simulink model "soc_dvbs2_fpga"  (R2025b)
settings: Solver=FixedStepDiscrete  StartTime=0.0  StopTime=0  RelTol=1e-3
InitFcn:
  | soc_dvbs2_init;
values from neighbouring files (symbols this model uses):
  Rsym = 4e6    (= 4000000)    [soc_dvbs2_init.m]
  soc_dvbs2_txPacketBits = [1 1 0 1 0 1 1 1 0 1 1 1 ... (2972 elements, 2972x1)]    [soc_dvbs2_txPacketBits.mat]
  syncWord = (dec2bin(hex2dec('AC')) - '0').'    [soc_dvbs2_init.m]
  txDataOut = txobj(frameBits(:))    [soc_dvbs2_init.m]
  txFiltCoeff = txobj.pTxFilterCoeff    [soc_dvbs2_init.m]
undefined symbols (not defined in the file or in its folder): Add, coefficientsLog, coefficientsSqrt1, coefficientsSqrt2, dataBits, designMultirateFIR, noisePow, NumBits1, NumBits2, seedsURNG1, seedsURNG2, Shift, Slope1, Slope2, soc_dvbs2_designFIRFilter, txDataOutS1, txDataOutS10, txDataOutS12, txDataOutS13, txDataOutS14, txDataOutS15, txDataOutS16, txDataOutS18, txDataOutS19, txDataOutS2, txDataOutS20, txDataOutS21, txDataOutS22, txDataOutS24, txDataOutS25, txDataOutS26, txDataOutS27, txDataOutS3, txDataOutS4, txDataOutS5, txDataOutS6, txDataOutS7, txDataOutS8, txDataOutS9
libraries: simulink x214, hdlsllib x211, dspsigops x22, dsphdlfiltering2 x8, dsphdlsigops2 x5, commseqgen3 x5, dsphdlmathfun2 x3, hwlogicconnlib x2, whdledac x2, commhdlcrc x2, whdlutilities x1, whdlmod x1
(part 4 of 12)

== system soc_dvbs2_fpga/DVBS2/DVBS2 TxRx/DVB-S2 HDL Receiver/Synchronizer and PL Header Decoder/Fine Phase Synchronizer/Direct Digital Synthesis ==
  v : Inport
  rst : Inport  Port=2
  Constant : Constant  Value=true  SampleTime=-1
  Constant1 : Constant  Value=FPCV  OutDataTypeStr=boolean  SampleTime=-1
  Constant2 : Constant  Value=complex(1)  OutDataTypeStr=Inherit: Inherit via back propagation  SampleTime=-1
  Data Type Conversion : DataTypeConversion  OutDataTypeStr=fixdt(1,21,21)  SaturateOnIntegerOverflow=off  RndMeth=Floor
  Data Type Conversion1 : DataTypeConversion  OutDataTypeStr=fixdt(1,21,0)  ConvertRealWorld=Stored Integer (SI)  SaturateOnIntegerOverflow=off  RndMeth=Floor
  Delay1 : Delay  DelayLength=1
  Delay12 : Delay  DelayLength=1
  Multiport Switch : MultiPortSwitch  DataPortOrder=Zero-based contiguous  Inputs=2  zeroidx=on  SaturateOnIntegerOverflow=off  InputSameDT=off
  NCO HDL Optimized : dsphdlsigops2/NCO  PhaseIncrementSource=Property  PhaseIncrement=0  PhaseOffsetSource=Input port  PhaseOffset=0  DitherSource=None  NumDitherBits=4  SamplesPerFrame=1  LUTCompress=off  ResetAction=on  Waveform=Complex exponential  PhasePort=off  SimulateUsing=Code generation  AccumulatorWL=21  PhaseQuantization=on  NumQuantizerAccumulatorBits=14  OutputDataType=Binary point scaling  OutputWL=16  OutputFL=14
  Terminator : Terminator
  xph : Outport
  wires:
  rst/1 -> NCO HDL Optimized/2
  Multiport Switch/1 -> Delay1/1
  Constant2/1 -> Multiport Switch/2
  Constant1/1 -> Multiport Switch/1
  Delay1/1 -> xph/1
  Delay12/1 -> Data Type Conversion/1
  NCO HDL Optimized/2 -> Terminator/1
  Constant/1 -> NCO HDL Optimized/3
  NCO HDL Optimized/1 -> Multiport Switch/3
  Data Type Conversion1/1 -> NCO HDL Optimized/1
  Data Type Conversion/1 -> Data Type Conversion1/1
  v/1 -> Delay12/1

== system soc_dvbs2_fpga/DVBS2/DVBS2 TxRx/DVB-S2 HDL Receiver/Synchronizer and PL Header Decoder/Fine Phase Synchronizer/Loop Filter ==
  e : Inport
  En : Inport  Port=2
  rst : Inport  Port=3
  Add : Sum  Inputs=|++  OutDataTypeStr=Inherit: Same as first input
  Delay1 : Delay
  Delay12 : Delay
  Gain : Gain  Gain=fi(config.FPCLoopFilterIntegGain/(2*pi),0,16)  ParamDataTypeStr=Inherit: Inherit from 'Gain'  OutDataTypeStr=fixdt(1,21,21)
  Unit Delay Enabled Resettable Synchronous : hdlsllib/Discrete/Unit Delay Enabled Resettable Synchronous  InitialCondition=0.0  SampleTime=-1
  v : Outport
  rstOut : Outport  Port=2
  wires:
  rst/1 -> Unit Delay Enabled Resettable Synchronous/3, rstOut/1
  En/1 -> Unit Delay Enabled Resettable Synchronous/2
  Delay1/1 -> Gain/1
  Delay12/1 -> Add/1
  Unit Delay Enabled Resettable Synchronous/1 -> v/1, Add/2
  Add/1 -> Unit Delay Enabled Resettable Synchronous/1
  Gain/1 -> Delay12/1
  e/1 -> Delay1/1

== system soc_dvbs2_fpga/DVBS2/DVBS2 TxRx/DVB-S2 HDL Receiver/Synchronizer and PL Header Decoder/Fine Phase Synchronizer/Phase Error Detector ==
  dataIn : Inport
  Compare To Constant : simulink/Logic and Bit Operations/Compare To Constant  relop=>=  const=0  OutDataTypeStr=boolean
  Compare To Constant1 : simulink/Logic and Bit Operations/Compare To Constant  relop=>=  const=0  OutDataTypeStr=boolean
  Complex to Real-Imag : ComplexToRealImag
  Complex to Real-Imag1 : ComplexToRealImag  Output=Imag
  Constant : Constant  OutDataTypeStr=fixdt(1,2,0)  SampleTime=-1
  Constant1 : Constant  Value=-1  OutDataTypeStr=fixdt(1,2,0)  SampleTime=-1
  Constant2 : Constant  OutDataTypeStr=fixdt(1,2,0)  SampleTime=-1
  Delay{1..5,12} (6 alike) : Delay  DelayLength=1
  Delay6 : Delay
  Delay7 : Delay
  Delay8 : Delay
  Product : Product  OutDataTypeStr=Inherit: Same as first input
  Real-Imag to Complex : RealImagToComplex
  Switch : Switch  Criteria=u2 ~= 0  SaturateOnIntegerOverflow=off  InputSameDT=off
  Switch1 : Switch  Criteria=u2 ~= 0  SaturateOnIntegerOverflow=off  InputSameDT=off
  e : Outport
  wires:
  Delay8/1 -> Complex to Real-Imag1/1
  Delay7/1 -> Product/2
  Delay6/1 -> Product/1
  Delay5/1 -> Delay6/1
  Delay4/1 -> Real-Imag to Complex/2
  Delay3/1 -> Real-Imag to Complex/1
  Delay2/1 -> Compare To Constant1/1
  Delay1/1 -> Delay5/1
  Delay12/1 -> Compare To Constant/1
  Complex to Real-Imag1/1 -> e/1
  Product/1 -> Delay8/1
  dataIn/1 -> Complex to Real-Imag/1, Delay1/1
  Real-Imag to Complex/1 -> Delay7/1
  Switch1/1 -> Delay4/1
  Switch/1 -> Delay3/1
  Constant2/1 -> Switch1/3
  Constant1/1 -> Switch/3, Switch1/1
  Constant/1 -> Switch/1
  Compare To Constant1/1 -> Switch1/2
  Compare To Constant/1 -> Switch/2
  Complex to Real-Imag/2 -> Delay2/1
  Complex to Real-Imag/1 -> Delay12/1

== system soc_dvbs2_fpga/DVBS2/DVBS2 TxRx/DVB-S2 HDL Receiver/Synchronizer and PL Header Decoder/Fine Phase Synchronizer/Power Q and Beta Offset Rotation ==
  dataIn : Inport
  mod : Inport  Port=2
  Complex Multiplier : Subsystem  VariantControl=Use 3 multipliers and 5 adders
      mask Display: disp(['Complex Multiplier' newline 'Latency = 7']);
  Complex Multiplier1 : Subsystem  VariantControl=Use 3 multipliers and 5 adders
      mask Display: disp(['Complex Multiplier' newline 'Latency = 7']);
  Complex Multiplier2 : Subsystem  VariantControl=Use 3 multipliers and 5 adders
      mask Display: disp(['Complex Multiplier' newline 'Latency = 7']);
  Delay{1..3,5,7,9..12,24..27,36} (14 alike) : Delay  DelayLength=1
  Delay{4,6,8,13..20} (11 alike) : Delay  DelayLength=7
  Delay{28..35} (8 alike) : Delay
  Gain : Subsystem  VariantControl=Use 3 multipliers and 5 adders
      mask Display: disp(['Rotate by pi/4' newline 'Latency = 7']);
  Gain1 : Subsystem  VariantControl=Use 3 multipliers and 5 adders
      mask Display: disp(['Rotate by pi/4' newline 'Latency = 7']);
  Multiport Switch : MultiPortSwitch  DataPortOrder=Zero-based contiguous  Inputs=4  zeroidx=on  SaturateOnIntegerOverflow=off  InputSameDT=off
  dataOut : Outport
  wires:
  Delay20/1 -> Delay30/1
  Delay19/1 -> Delay28/1
  Delay36/1 -> dataOut/1
  Delay15/1 -> Delay26/1
  Delay14/1 -> Delay25/1
  Delay13/1 -> Delay24/1
  Delay12/1 -> Complex Multiplier2/2(In2)
  Delay2/1 -> Complex Multiplier1/1(In1)
  Complex Multiplier1/1(Out1) -> Delay10/1
  Delay5/1 -> Complex Multiplier1/2(In2)
  Complex Multiplier/1(Out1) -> Delay2/1, Delay1/1
  mod/1 -> Multiport Switch/1
  Delay35/1 -> Gain1/1(In1)
  Delay34/1 -> Delay20/1
  Delay33/1 -> Gain/1(In1)
  Delay32/1 -> Delay19/1
  Delay31/1 -> Multiport Switch/5
  Delay30/1 -> Multiport Switch/4
  Delay29/1 -> Multiport Switch/3
  Delay28/1 -> Multiport Switch/2
  Delay27/1 -> Delay35/1
  Delay26/1 -> Delay34/1
  Delay25/1 -> Delay33/1
  Delay24/1 -> Delay32/1
  Delay11/1 -> Delay13/1
  Delay9/1 -> Delay14/1
  Delay10/1 -> Delay15/1, Complex Multiplier2/1(In1)
  Delay18/1 -> Delay12/1
  Delay17/1 -> Delay11/1
  Delay16/1 -> Delay9/1
  Delay8/1 -> Delay7/1
  Delay6/1 -> Delay5/1
  Delay4/1 -> Delay3/1
  Delay7/1 -> Delay18/1
  Delay3/1 -> Delay17/1
  Delay1/1 -> Delay16/1
  dataIn/1 -> Delay8/1, Delay6/1, Complex Multiplier/2(In2), Complex Multiplier/1(In1), Delay4/1
  Multiport Switch/1 -> Delay36/1
  Gain/1(Out1) -> Delay29/1
  Gain1/1(Out1) -> Delay31/1
  Complex Multiplier2/1(Out1) -> Delay27/1

== system soc_dvbs2_fpga/DVBS2/DVBS2 TxRx/DVB-S2 HDL Receiver/Synchronizer and PL Header Decoder/PL Header Recovery/No HDL ==
  has Pilots : Inport
  Enable : EnablePort
  To Workspace : ToWorkspace  VariableName=simHasPilots  SaveFormat=Timeseries  SampleTime=-1
      settings: Save2DSignal=2-D array (concatenate along first dimension)
  wires:
  has Pilots/1 -> To Workspace/1

== system soc_dvbs2_fpga/DVBS2/DVBS2 TxRx/DVB-S2 HDL Receiver/Synchronizer and PL Header Decoder/PL Header Recovery/No HDL1 ==
  valid : Inport
  endOfPLSc : Inport  Port=2
  Bias : Bias  Bias=1  SaturateOnIntegerOverflow=off
  Data Type Conversion : DataTypeConversion  OutDataTypeStr=double  SaturateOnIntegerOverflow=off  RndMeth=Floor
  HDL Counter : hdlsllib/Sources/HDL Counter  CountType=Free running  CountInit=0  CountStep=1  CountMax=25  CountFromType=Initial value  CountFrom=0  CountResetPort=off  CountLoadPort=off  CountEnbPort=on  CountDirPort=off  CountHitOutputPort=off  CountDataType=Unsigned  CountWordLen=32  CountFracLen=0  CountSampTime=1
  Subsystem : Subsystem
  wires:
  endOfPLSc/1 -> Subsystem/Enable
  Bias/1 -> Subsystem/1(In1)
  valid/1 -> HDL Counter/1
  Data Type Conversion/1 -> Bias/1
  HDL Counter/1 -> Data Type Conversion/1

== system soc_dvbs2_fpga/DVBS2/DVBS2 TxRx/DVB-S2 HDL Receiver/Synchronizer and PL Header Decoder/PL Header Recovery/PL Frame Demultiplexer ==
  endOfSOFIn : Inport
  validIn : Inport  Port=2
  Compare To Constant : simulink/Logic and Bit Operations/Compare To Constant  relop=<=  const=config.PLSCLength - 1  OutDataTypeStr=boolean
  Delay : Delay  DelayLength=64
  Delay{1..3,5..8,10..13} (11 alike) : Delay  DelayLength=1
  HDL Counter : hdlsllib/Sources/HDL Counter  CountType=Free running  CountInit=0  CountStep=1  CountMax=25  CountFromType=Initial value  CountFrom=0  CountResetPort=on  CountLoadPort=off  CountEnbPort=on  CountDirPort=off  CountHitOutputPort=off  CountDataType=Unsigned  CountWordLen=32  CountFracLen=0  CountSampTime=1
  Logical Operator : Logic  Inputs=3  AllPortsSameDT=off  OutDataTypeStr=boolean
  Logical Operator1 : Logic  AllPortsSameDT=off  OutDataTypeStr=boolean
  Logical Operator2 : Logic  Operator=NOT  AllPortsSameDT=off  OutDataTypeStr=boolean
  Unit Delay Enabled Synchronous : hdlsllib/Discrete/Unit Delay Enabled Synchronous  InitialCondition=0.0  SampleTime=-1
  hValid : Outport
  dValid : Outport  Port=2
  endOfPLSC : Outport  Port=3
  wires:
  Delay/1 -> Delay5/1
  Delay13/1 -> endOfPLSC/1
  Delay12/1 -> dValid/1
  Delay11/1 -> hValid/1
  Delay8/1 -> Logical Operator1/2
  Delay7/1 -> Delay11/1
  Delay6/1 -> Logical Operator2/1
  Delay5/1 -> Delay10/1
  Delay2/1 -> Logical Operator/3, Delay8/1
  Delay1/1 -> Logical Operator/2
  Delay3/1 -> Logical Operator/1
  Delay10/1 -> Delay13/1
  HDL Counter/1 -> Compare To Constant/1
  Logical Operator1/1 -> Delay12/1
  Logical Operator2/1 -> Logical Operator1/1
  Unit Delay Enabled Synchronous/1 -> Delay3/1
  Compare To Constant/1 -> Delay1/1
  Logical Operator/1 -> Delay7/1, Delay6/1
  validIn/1 -> HDL Counter/2, Delay2/1
  endOfSOFIn/1 -> Unit Delay Enabled Synchronous/1, Delay/1, Unit Delay Enabled Synchronous/2, HDL Counter/1

== system soc_dvbs2_fpga/DVBS2/DVBS2 TxRx/DVB-S2 HDL Receiver/Synchronizer and PL Header Decoder/PL Header Recovery/PL Header Decoder ==
  dataIn : Inport
  hasPilots : Inport  Port=2
  endOfSOF : Inport  Port=3
  validIn : Inport  Port=4
  Bit Flipping and Averaging : Subsystem
  Constant : Constant  Value=complex(0)  OutDataTypeStr=Inherit: Inherit via back propagation  SampleTime=-1
  Delay{1..4} (4 alike) : Delay  DelayLength=1
  Delay5 : Delay  DelayLength=10
  Delay6 : Delay  DelayLength=4
  Extract Bits2 : simulink/Logic and Bit Operations/Extract Bits  bitsToExtract=Range of bits  numBits=8  bitIdxRange=[1 5]  outScalingMode=Treat bit field as an integer
  Extract Bits3 : simulink/Logic and Bit Operations/Extract Bits  bitsToExtract=Range of bits  numBits=8  bitIdxRange=0  outScalingMode=Treat bit field as an integer
  ML Decoder : Subsystem
  PLSC Descrambler : Subsystem
  Switch : Switch  Criteria=u2 ~= 0  SaturateOnIntegerOverflow=off  InputSameDT=off
  pi/2 BPSK Soft Bit Generator : Subsystem
  modcod : Outport
  FECFrame : Outport  Port=2
  wires:
  Delay6/1 -> Bit Flipping and Averaging/5(hasPilots)
  Delay5/1 -> Delay6/1
  Delay4/1 -> Delay5/1
  Delay2/1 -> PLSC Descrambler/3(validIn), Switch/2
  Delay1/1 -> PLSC Descrambler/2(resetIn)
  Delay3/1 -> Switch/1
  Bit Flipping and Averaging/3(resetOut) -> ML Decoder/3(reset)
  pi/2 BPSK Soft Bit Generator/4(resetOut) -> Bit Flipping and Averaging/4(resetIn)
  PLSC Descrambler/4(resetOut) -> pi/2 BPSK Soft Bit Generator/4(resetIn)
  Extract Bits2/1 -> modcod/1
  Extract Bits3/1 -> FECFrame/1
  ML Decoder/1(bits6Out) -> Extract Bits2/1, Extract Bits3/1
  Bit Flipping and Averaging/2(validOut) -> ML Decoder/2(PLSCValid32)
  PLSC Descrambler/3(validOut) -> pi/2 BPSK Soft Bit Generator/3(validIn)
  pi/2 BPSK Soft Bit Generator/3(validOut) -> Bit Flipping and Averaging/3(validIn)
  hasPilots/1 -> Delay4/1
  pi/2 BPSK Soft Bit Generator/2(indexIndicatorOut) -> Bit Flipping and Averaging/2(indexIndicater)
  Bit Flipping and Averaging/1(dataOut) -> ML Decoder/1(dataIn)
  Switch/1 -> PLSC Descrambler/1(dataIn)
  Constant/1 -> Switch/3
  PLSC Descrambler/2(indexIndicator) -> pi/2 BPSK Soft Bit Generator/2(indexIndicatorIn)
  PLSC Descrambler/1(dataOut) -> pi/2 BPSK Soft Bit Generator/1(dataIn)
  pi/2 BPSK Soft Bit Generator/1(dataOut) -> Bit Flipping and Averaging/1(dataIn)
  endOfSOF/1 -> Delay1/1
  dataIn/1 -> Delay3/1
  validIn/1 -> Delay2/1

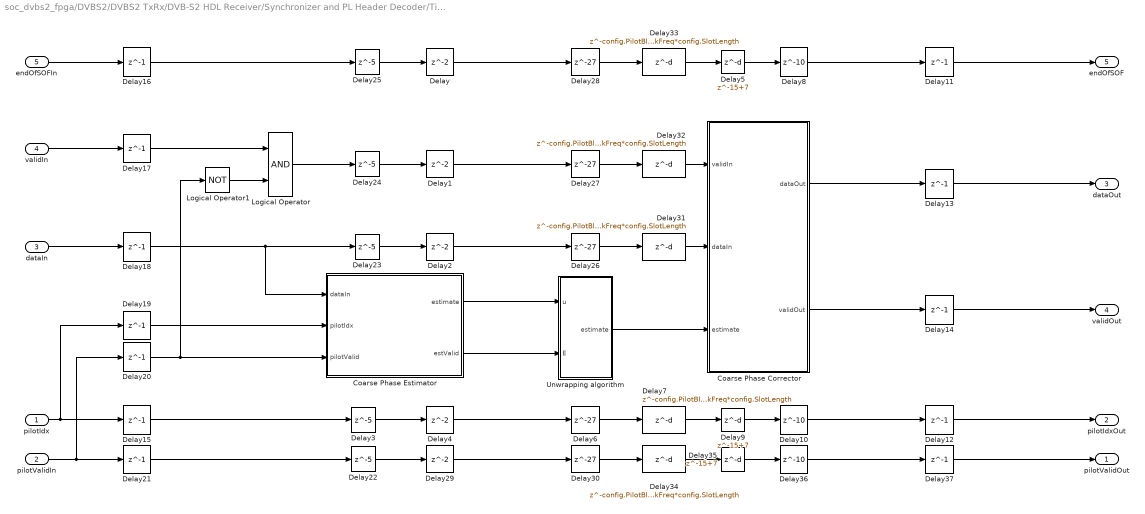
== system soc_dvbs2_fpga/DVBS2/DVBS2 TxRx/DVB-S2 HDL Receiver/Synchronizer and PL Header Decoder/Time Frequency and Coarse Phase Synchronizer/Coarse Phase Synchronizer ==
  pilotIdx : Inport
  pilotValidIn : Inport  Port=2
  dataIn : Inport  Port=3
  validIn : Inport  Port=4
  endOfSOFIn : Inport  Port=5
  Coarse Phase Corrector : Subsystem
  Coarse Phase Estimator : Subsystem
  Delay{,1..2,4,29} (5 alike) : Delay
  Delay10 : Delay  DelayLength=10  InitialCondition=0
  Delay{11..21,37} (12 alike) : Delay  DelayLength=1  InitialCondition=0
  Delay{3,22..25} (5 alike) : Delay  DelayLength=5  InitialCondition=0
  Delay{6,26..28,30} (5 alike) : Delay  DelayLength=27
  Delay{7,31..34} (5 alike) : Delay  DelayLength=config.PilotBlkFreq*config.SlotLength
  Delay35 : Delay  DelayLength=15+7
  Delay36 : Delay  DelayLength=10  InitialCondition=0
  Delay5 : Delay  DelayLength=15+7
  Delay8 : Delay  DelayLength=10  InitialCondition=0
  Delay9 : Delay  DelayLength=15+7
  Logical Operator : Logic  AllPortsSameDT=off  OutDataTypeStr=boolean
  Logical Operator1 : Logic  Operator=NOT  AllPortsSameDT=off  OutDataTypeStr=boolean
  Unwrapping algorithm : Subsystem
      mask init:
      | Simulink.suppressDiagnostic(gcb, 'SimulinkFixedPoint:util:Overflowoccurred');
  pilotValidOut : Outport
  pilotIdxOut : Outport  Port=2
  dataOut : Outport  Port=3
  validOut : Outport  Port=4
  endOfSOF : Outport  Port=5
  wires:
  Delay37/1 -> pilotValidOut/1
  Delay36/1 -> Delay37/1
  Delay35/1 -> Delay36/1
  Delay34/1 -> Delay35/1
  Delay30/1 -> Delay34/1
  Delay29/1 -> Delay30/1
  Delay22/1 -> Delay29/1
  Delay21/1 -> Delay22/1
  Delay15/1 -> Delay3/1
  Delay12/1 -> pilotIdxOut/1
  Delay10/1 -> Delay12/1
  Delay9/1 -> Delay10/1
  Delay7/1 -> Delay9/1
  Delay6/1 -> Delay7/1
  Delay4/1 -> Delay6/1
  Delay3/1 -> Delay4/1
  Logical Operator1/1 -> Logical Operator/2
  Delay17/1 -> Logical Operator/1
  Delay18/1 -> Delay23/1, Coarse Phase Estimator/1(dataIn)
  Coarse Phase Estimator/1(estimate) -> Unwrapping algorithm/1(u)
  Delay33/1 -> Delay5/1
  Delay32/1 -> Coarse Phase Corrector/1(validIn)
  Delay31/1 -> Coarse Phase Corrector/2(dataIn)
  Delay27/1 -> Delay32/1
  Unwrapping algorithm/1(estimate) -> Coarse Phase Corrector/3(estimate)
  Delay28/1 -> Delay33/1
  Delay26/1 -> Delay31/1
  Coarse Phase Estimator/2(estValid) -> Unwrapping algorithm/2(E)
  Coarse Phase Corrector/2(validOut) -> Delay14/1
  Coarse Phase Corrector/1(dataOut) -> Delay13/1
  Delay2/1 -> Delay26/1
  Delay25/1 -> Delay/1
  Delay24/1 -> Delay1/1
  Delay23/1 -> Delay2/1
  Delay20/1 -> Coarse Phase Estimator/3(pilotValid), Logical Operator1/1
  Delay19/1 -> Coarse Phase Estimator/2(pilotIdx)
  validIn/1 -> Delay17/1
  endOfSOFIn/1 -> Delay16/1
  Delay14/1 -> validOut/1
  Delay13/1 -> dataOut/1
  Delay11/1 -> endOfSOF/1
  Delay8/1 -> Delay11/1
  Delay5/1 -> Delay8/1
  pilotIdx/1 -> Delay15/1, Delay19/1
  pilotValidIn/1 -> Delay20/1, Delay21/1
  dataIn/1 -> Delay18/1
  Delay1/1 -> Delay27/1
  Delay/1 -> Delay28/1
  Logical Operator/1 -> Delay24/1
  Delay16/1 -> Delay25/1

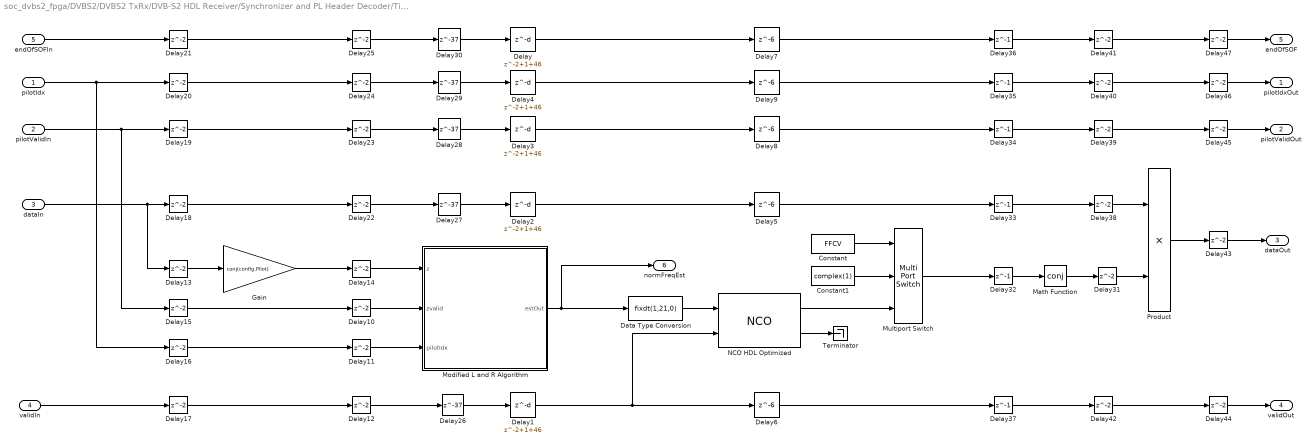
== system soc_dvbs2_fpga/DVBS2/DVBS2 TxRx/DVB-S2 HDL Receiver/Synchronizer and PL Header Decoder/Time Frequency and Coarse Phase Synchronizer/Fine Frequency Synchronizer ==
  pilotIdx : Inport
  pilotValidIn : Inport  Port=2
  dataIn : Inport  Port=3
  validIn : Inport  Port=4
  endOfSOFIn : Inport  Port=5
  Constant : Constant  Value=FFCV  OutDataTypeStr=boolean  SampleTime=-1
  Constant1 : Constant  Value=complex(1)  OutDataTypeStr=Inherit: Inherit via back propagation  SampleTime=-1
  Data Type Conversion : DataTypeConversion  OutDataTypeStr=fixdt(1,21,0)  ConvertRealWorld=Stored Integer (SI)  SaturateOnIntegerOverflow=off  RndMeth=Floor
  Delay{,1..4} (5 alike) : Delay  DelayLength=2+1+46
  Delay{10..25,31,38..47} (27 alike) : Delay
  Delay{26..30} (5 alike) : Delay  DelayLength=37
  Delay{32..37} (6 alike) : Delay  DelayLength=1
  Delay{5..9} (5 alike) : Delay  DelayLength=6
  Gain : Gain  Gain=conj(config.Pilot)  OutDataTypeStr=Inherit: Same as input
      mask init:
      | Simulink.suppressDiagnostic(gcb, 'SimulinkFixedPoint:util:fxpParameterPrecisionLoss');
  Math Function : Math  Operator=conj
  Modified L and R Algorithm : Subsystem
  Multiport Switch : MultiPortSwitch  DataPortOrder=Zero-based contiguous  Inputs=2  zeroidx=on  SaturateOnIntegerOverflow=off  InputSameDT=off
  NCO HDL Optimized : dsphdlsigops2/NCO  PhaseIncrementSource=Input port  PhaseIncrement=100  PhaseOffsetSource=Property  PhaseOffset=0  DitherSource=None  NumDitherBits=4  SamplesPerFrame=1  LUTCompress=off  ResetAction=off  Waveform=Complex exponential  PhasePort=off  SimulateUsing=Code generation  AccumulatorWL=21  PhaseQuantization=on  NumQuantizerAccumulatorBits=14  OutputDataType=Binary point scaling  OutputWL=16  OutputFL=14
  Product : Product  OutDataTypeStr=Inherit: Same as first input
  Terminator : Terminator
  pilotIdxOut : Outport
  pilotValidOut : Outport  Port=2
  dataOut : Outport  Port=3
  validOut : Outport  Port=4
  endOfSOF : Outport  Port=5
  normFreqEst : Outport  Port=6
  wires:
  Multiport Switch/1 -> Delay32/1
  Constant1/1 -> Multiport Switch/2
  Constant/1 -> Multiport Switch/1
  Modified L and R Algorithm/1(estOut) -> normFreqEst/1, Data Type Conversion/1
  dataIn/1 -> Delay18/1, Delay13/1
  Delay47/1 -> endOfSOF/1
  Delay46/1 -> pilotIdxOut/1
  Delay45/1 -> pilotValidOut/1
  Delay44/1 -> validOut/1
  Delay43/1 -> dataOut/1
  Delay42/1 -> Delay44/1
  Delay41/1 -> Delay47/1
  Delay40/1 -> Delay46/1
  Delay39/1 -> Delay45/1
  Delay38/1 -> Product/1
  Delay31/1 -> Product/2
  Delay37/1 -> Delay42/1
  Delay36/1 -> Delay41/1
  Delay35/1 -> Delay40/1
  Delay34/1 -> Delay39/1
  Delay33/1 -> Delay38/1
  Delay32/1 -> Math Function/1
  Delay30/1 -> Delay/1
  Delay29/1 -> Delay4/1
  Delay28/1 -> Delay3/1
  Delay27/1 -> Delay2/1
  Delay26/1 -> Delay1/1
  Delay25/1 -> Delay30/1
  Delay24/1 -> Delay29/1
  Delay23/1 -> Delay28/1
  Delay22/1 -> Delay27/1
  Delay21/1 -> Delay25/1
  Delay20/1 -> Delay24/1
  Delay19/1 -> Delay23/1
  Delay18/1 -> Delay22/1
  Delay17/1 -> Delay12/1
  Delay16/1 -> Delay11/1
  Delay15/1 -> Delay10/1
  Delay13/1 -> Gain/1
  Delay12/1 -> Delay26/1
  Delay11/1 -> Modified L and R Algorithm/3(pilotIdx)
  Delay10/1 -> Modified L and R Algorithm/2(zvalid)
  Delay14/1 -> Modified L and R Algorithm/1(z)
  Math Function/1 -> Delay31/1
  NCO HDL Optimized/2 -> Terminator/1
  Delay6/1 -> Delay37/1
  Delay1/1 -> NCO HDL Optimized/2, Delay6/1
  NCO HDL Optimized/1 -> Multiport Switch/3
  Product/1 -> Delay43/1
  Data Type Conversion/1 -> NCO HDL Optimized/1
  Delay9/1 -> Delay35/1
  Delay8/1 -> Delay34/1
  Delay7/1 -> Delay36/1
  Delay5/1 -> Delay33/1
  Delay4/1 -> Delay9/1
  Delay3/1 -> Delay8/1
  Delay2/1 -> Delay5/1
  Delay/1 -> Delay7/1
  Gain/1 -> Delay14/1
  pilotValidIn/1 -> Delay15/1, Delay19/1
  pilotIdx/1 -> Delay16/1, Delay20/1
  validIn/1 -> Delay17/1
  endOfSOFIn/1 -> Delay21/1

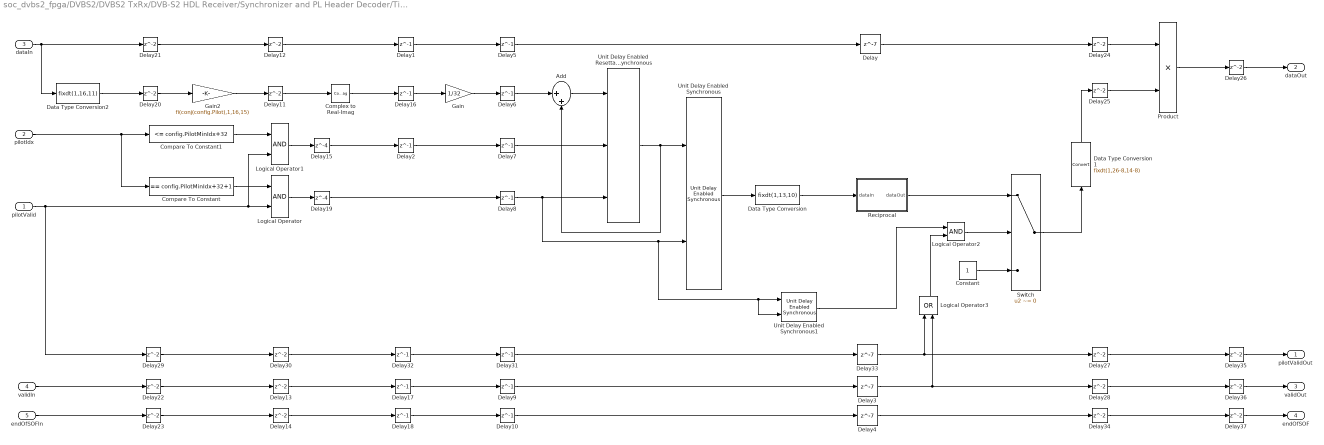
== system soc_dvbs2_fpga/DVBS2/DVBS2 TxRx/DVB-S2 HDL Receiver/Synchronizer and PL Header Decoder/Time Frequency and Coarse Phase Synchronizer/Fine Gain Control ==
  pilotValid : Inport
  pilotIdx : Inport  Port=2
  dataIn : Inport  Port=3
  validIn : Inport  Port=4
  endOfSOFIn : Inport  Port=5
  Add : Sum  Inputs=|++  OutDataTypeStr=Inherit: Same as first input
  Compare To Constant : simulink/Logic and Bit Operations/Compare To Constant  relop===  const=config.PilotMinIdx+32+1  OutDataTypeStr=boolean
  Compare To Constant1 : simulink/Logic and Bit Operations/Compare To Constant  relop=<=  const=config.PilotMinIdx+32  OutDataTypeStr=boolean
  Complex to Real-Imag : ComplexToRealImag  Output=Real
  Constant : Constant  OutDataTypeStr=Inherit: Inherit via back propagation  SampleTime=-1
  Data Type Conversion : DataTypeConversion  OutDataTypeStr=fixdt(1,13,10)  SaturateOnIntegerOverflow=off  RndMeth=Floor
  Data Type Conversion1 : DataTypeConversion  OutDataTypeStr=fixdt(1,26-8,14-8)  SaturateOnIntegerOverflow=off  RndMeth=Floor
  Data Type Conversion2 : DataTypeConversion  OutDataTypeStr=fixdt(1,16,11)  SaturateOnIntegerOverflow=off  RndMeth=Floor
  Delay{,3..4,33} (4 alike) : Delay  DelayLength=7
  Delay{1..2,5..10,16..18,31..32} (13 alike) : Delay  DelayLength=1
  Delay{11..14,20..30,34..37} (19 alike) : Delay
  Delay15 : Delay  DelayLength=4
  Delay19 : Delay  DelayLength=4
  Gain : Gain  Gain=1/32  ParamDataTypeStr=fixdt(0,5,5)  OutDataTypeStr=Inherit: Same as input
  Gain2 : Gain  Gain=fi(conj(config.Pilot),1,16,15)  ParamDataTypeStr=Inherit: Inherit from 'Gain'  OutDataTypeStr=Inherit: Same as input
  Logical Operator : Logic  AllPortsSameDT=off  OutDataTypeStr=boolean
  Logical Operator1 : Logic  AllPortsSameDT=off  OutDataTypeStr=boolean
  Logical Operator2 : Logic  AllPortsSameDT=off  OutDataTypeStr=boolean
  Logical Operator3 : Logic  Operator=OR  AllPortsSameDT=off  OutDataTypeStr=boolean
  Product : Product  OutDataTypeStr=Inherit: Same as first input
  Reciprocal : Subsystem  mask{WL=13, FL=10, outWL=26, Mapp=RAM - Based}
      mask prompts: WL "Input Word Length :"; FL "Input Fractional Length :"; outWL "Output Word Length :"; Mapp "Mapping Type:"
      mask init:
      | % Inverse for 18 bit numbers: partitioned into 3+15 bits. 2^3 LUTs with 2^15
      | % combinations will store a total of 2^18 combinations.
      | % As each LUT has 2^15 combinations the data type of output has a maximum
      | % limit of 32 bits (2^20 is a maximum number of bits an LUT can store)
      | 
      | % Non tunable Parameters
      | % FL = 16;
      | % outWL = 31;
      | % WL = 18;
      | % This Parameter is not given for mask
      | LUTAddrWL = WL - 1; % this will implement 2 LUTs
      | 
      | % validate Non tunable parameters
      | % condition for validation: 2^20 bits is the maximum number of bits an LUT can store
      | if LUTAddrWL >= 20   % As 2^20 is the limit
      |     error('invalid LUTAddrWL');
      | end
      | if outWL >= 2^(20-LUTAddrWL)  % 2^(20-LUTAddrWL) is the maximum outWL based on condition for validation
      |     error('invalid outWL')
      | end
      | 
      | % calculate number of LUTs required
      | muxSelectorWL = WL - LUTAddrWL;
      | nLUT = 2^muxSelectorWL;
      | 
      | % Generate all possible RWV inputs using WL and FL
      | allInputRangeSI = -2^(WL-1):2^(WL-1)-1;  % as a stored integer
      | allInputRWV = allInputRangeSI * 2^(-FL);
      | 
      | % define the function for all the RWV input
      | reciprocal = 1./allInputRWV;
      | 
      | % store the function output in LUT
      | allLUTAddr = (0:2^LUTAddrWL-1);
      | LUT = zeros(length(allLUTAddr),nLUT);
      | for i = 0:nLUT-1
      |     LUT(:,i+1) = reciprocal(i*2^LUTAddrWL+1:(i+1)*2^LUTAddrWL);
      | end
      | 
      | % quantize the function with outWL
      | NT = numerictype(fi(LUT(abs(LUT) ~= inf),1,outWL)); % inf and -inf will be quantized with max and min values with NT data type
      | if NT.WordLength < NT. FractionLength
      |     NT.FractionLength = NT.WordLength
      | end
      | LUT = fi(LUT,NT,'RoundingMethod','Nearest');
      | 
      | paths = find_system([gcb '/Function Impl'],'BlockType','Delay');
      | 
      | for i = 1:length(paths)
      |     if Mapp == 1
      |         hdlset_param(paths{i},'ResetType','default');
      |     else
      |         hdlset_param(paths{i},'ResetType','none');
      |     end
      | end
      mask TypeOptions Mapp: LUT - Based | RAM - Based
      mask DialogControl DescGroupVar Prompt: LUT - Based function
      mask DialogControl DescTextVar Prompt: This block is implemented for real reciprocal
      mask Display: disp(['Reciprocal\n' get_param(gcb,'Mapp') '\nLatency = 7'])
  Switch : Switch  Criteria=u2 ~= 0  SaturateOnIntegerOverflow=off  InputSameDT=off
  Unit Delay Enabled Synchronous : hdlsllib/Discrete/Unit Delay Enabled Synchronous  InitialCondition=0.0  SampleTime=-1
  Unit Delay Enabled Synchronous1 : hdlsllib/Discrete/Unit Delay Enabled Synchronous  InitialCondition=0.0  SampleTime=-1
  Unit Delay Enabled Resettable Synchronous : hdlsllib/Discrete/Unit Delay Enabled Resettable Synchronous  InitialCondition=0.0  SampleTime=-1
  pilotValidOut : Outport
  dataOut : Outport  Port=2
  validOut : Outport  Port=3
  endOfSOF : Outport  Port=4
  wires:
  Data Type Conversion2/1 -> Delay20/1
  Data Type Conversion1/1 -> Delay25/1
  Delay27/1 -> Delay35/1
  Switch/1 -> Data Type Conversion1/1
  Logical Operator2/1 -> Switch/2
  Delay37/1 -> endOfSOF/1
  Delay36/1 -> validOut/1
  Delay35/1 -> pilotValidOut/1
  Delay34/1 -> Delay37/1
  Delay28/1 -> Delay36/1
  Delay26/1 -> dataOut/1
  Delay25/1 -> Product/2
  Delay24/1 -> Product/1
  Unit Delay Enabled Synchronous/1 -> Data Type Conversion/1
  Logical Operator3/1 -> Logical Operator2/2
  Complex to Real-Imag/1 -> Delay16/1
  Delay8/1 -> Unit Delay Enabled Resettable Synchronous/3, Unit Delay Enabled Synchronous/2, Unit Delay Enabled Synchronous1/1, Unit Delay Enabled Synchronous1/2
  Reciprocal/1(dataOut) -> Switch/1
  Unit Delay Enabled Synchronous1/1 -> Logical Operator2/1
  Constant/1 -> Switch/3
  Delay33/1 -> Logical Operator3/1, Delay27/1
  Delay32/1 -> Delay31/1
  Delay31/1 -> Delay33/1
  Delay30/1 -> Delay32/1
  Delay29/1 -> Delay30/1
  Delay23/1 -> Delay14/1
  Delay22/1 -> Delay13/1
  Delay21/1 -> Delay12/1
  Delay20/1 -> Gain2/1
  Delay19/1 -> Delay8/1
  Delay15/1 -> Delay2/1
  Delay14/1 -> Delay18/1
  Delay13/1 -> Delay17/1
  Delay12/1 -> Delay1/1
  Delay11/1 -> Complex to Real-Imag/1
  Delay10/1 -> Delay4/1
  Delay9/1 -> Delay3/1
  Delay7/1 -> Unit Delay Enabled Resettable Synchronous/2
  Delay6/1 -> Add/1
  Delay5/1 -> Delay/1
  Delay4/1 -> Delay34/1
  Delay3/1 -> Logical Operator3/2, Delay28/1
  Delay/1 -> Delay24/1
  Data Type Conversion/1 -> Reciprocal/1(dataIn)
  Product/1 -> Delay26/1
  Gain2/1 -> Delay11/1
  Delay1/1 -> Delay5/1
  Gain/1 -> Delay6/1
  Unit Delay Enabled Resettable Synchronous/1 -> Add/2, Unit Delay Enabled Synchronous/1
  Add/1 -> Unit Delay Enabled Resettable Synchronous/1
  Compare To Constant1/1 -> Logical Operator1/1
  Logical Operator1/1 -> Delay15/1
  Delay2/1 -> Delay7/1
  Logical Operator/1 -> Delay19/1
  Compare To Constant/1 -> Logical Operator/1
  Delay16/1 -> Gain/1
  pilotValid/1 -> Logical Operator1/2, Logical Operator/2, Delay29/1
  pilotIdx/1 -> Compare To Constant/1, Compare To Constant1/1
  Delay18/1 -> Delay10/1
  endOfSOFIn/1 -> Delay23/1
  validIn/1 -> Delay22/1
  dataIn/1 -> Data Type Conversion2/1, Delay21/1
  Delay17/1 -> Delay9/1

== system soc_dvbs2_fpga/DVBS2/DVBS2 TxRx/DVB-S2 HDL Receiver/Synchronizer and PL Header Decoder/Time Frequency and Coarse Phase Synchronizer/Pilot Blks Counter ==
  pilotIdx : Inport
  pilotValid : Inport  Port=2
  Compare To Constant : simulink/Logic and Bit Operations/Compare To Constant  relop===  const=config.PilotMinIdx  OutDataTypeStr=boolean
  Delay{1..4} (4 alike) : Delay  DelayLength=1
  HDL Counter : hdlsllib/Sources/HDL Counter  CountType=Free running  CountInit=0  CountStep=1  CountMax=25  CountFromType=Initial value  CountFrom=0  CountResetPort=off  CountLoadPort=off  CountEnbPort=on  CountDirPort=off  CountHitOutputPort=off  CountDataType=Unsigned  CountWordLen=16  CountFracLen=0  CountSampTime=1
  Logical Operator : Logic  AllPortsSameDT=off  OutDataTypeStr=boolean
  pilotBlkCount : Outport
  wires:
  Delay4/1 -> HDL Counter/1
  Delay3/1 -> pilotBlkCount/1
  Delay2/1 -> Logical Operator/2
  Delay1/1 -> Compare To Constant/1
  HDL Counter/1 -> Delay3/1
  pilotIdx/1 -> Delay1/1
  pilotValid/1 -> Delay2/1
  Compare To Constant/1 -> Logical Operator/1
  Logical Operator/1 -> Delay4/1

== system soc_dvbs2_fpga/DVBS2/DVBS2 TxRx/DVB-S2 HDL Receiver/Synchronizer and PL Header Decoder/Time Frequency and Coarse Phase Synchronizer/Time and Coarse Frequency Synchronizer ==
  note: Use this port to enable the CCFO
      | for higer carrier offsets
  dataIn : Inport
  validIn : Inport  Port=2
  Coarse Frequency Estimator : Subsystem
  Delay{1..4,7..9,14} (8 alike) : Delay
  Delay10 : Delay  DelayLength=1+1+1+14+4
  Delay11 : Delay  DelayLength=config.SOFLength
  Delay{5..6,28..32,34} (8 alike) : Delay  DelayLength=1
  Frame Synchronizer : Subsystem
      settings: PortSchema="{\"entries\":[{\"content\":{\"sides\":[{\"content\":{\"connectorIds\":[\"In1\",\"In2\"]},\"type\":\"ConnectorPlacement.EquallySpacedRectSide\",\"uuid\":\"07d09bb1-f07b-4fab-a4f2-f5b6f6f725b0\"},{\"content\":{\"connectorIds\":[\"Out1\",\"Out2\",\"Out3\",\"Out4\"],\"side\":\"RIGHT\"},\"type\":\"ConnectorPlacement.EquallySpacedRectSide\",\"uuid\":\"c1d2b5be-2891-4f3c-88c5-af394a100bb6\"},{\"content\":{\"connectorIds\":[\"Out5\"],\"side\":\"TOP\"},\"type\":\"ConnectorPlacement.EquallySpacedRectSide\",\"uuid\":\"10b34a60-aaa3-44cd-b5ea-a8382d3eca4e\"}]},\"type\":\"ConnectorPlacement.EquallySpacedConnector\",\"uuid\":\"75f7b276-e752-4165-bc1a-250d984d2b0b\"}],\"packageUris\":[\"http://schema.mathworks.com/mf0/Connector/R2020b\"],\"version\":\"1.0\"}"
  Math Function : Math  Operator=conj
  PL Data Descrambler and Pilot Valid Indicator : Subsystem
  Product : Product  OutDataTypeStr=Inherit: Same as first input
  RRC Receive Matched Filter : dsphdlfiltering2/Discrete FIR Filter  NumeratorSource=Property  Numerator=config.RRCImpulseResponse  NumeratorPrototype=[]  FilterStructure=Direct form systolic  SerializationOption=Minimum number of cycles between valid input samples  NumCycles=2  NumberOfMultipliers=2  SimulateUsing=Code generation  roundingMode=Floor  overflowMode=off  CoefficientsDataTypeStr=Inherit: Same word length as input  OutputDataTypeStr=Inherit: Same word length as input  ResetInputPort=off  HDLGlobalReset=off  CoeffMultiplier=Multiplier  UseMultForPow2Coeff=on  FrameInputSymmOptim=off
  Symbol Synchronizer : Subsystem
  rstCCFO : Constant  Value=true  SampleTime=-1
  VisualizeCorrelationSignals : Outport
  normCoarFreqEst : Outport  Port=2
  symbSyncDataOut : Outport  Port=3
  symbSyncValidOut : Outport  Port=4
  pilotIdx : Outport  Port=5
  pilotValid : Outport  Port=6
  dataOut : Outport  Port=7
  validOut : Outport  Port=8
  endOfSOF : Outport  Port=9
  hasPilots : Outport  Port=10
  wires:
  Delay34/1 -> hasPilots/1
  Delay32/1 -> endOfSOF/1
  PL Data Descrambler and Pilot Valid Indicator/5(endOfSOF) -> Delay32/1
  Delay4/1 -> RRC Receive Matched Filter/2
  Math Function/1 -> Delay5/1
  PL Data Descrambler and Pilot Valid Indicator/1(pilotidx) -> Delay28/1
  PL Data Descrambler and Pilot Valid Indicator/3(dataOut) -> Delay30/1
  Frame Synchronizer/2(validOut) -> PL Data Descrambler and Pilot Valid Indicator/2(validIn)
  Frame Synchronizer/3(endOfSOF) -> PL Data Descrambler and Pilot Valid Indicator/3(endOfSOFIn)
  Delay7/1 -> Coarse Frequency Estimator/2(dataIn)
  Delay30/1 -> Delay7/1, dataOut/1
  Coarse Frequency Estimator/2(normFreqEst) -> normCoarFreqEst/1
  Symbol Synchronizer/1(dataOut) -> symbSyncDataOut/1, Frame Synchronizer/1(dataIn)
  Delay31/1 -> validOut/1
  Coarse Frequency Estimator/1(complexEstimate) -> Delay6/1
  Delay28/1 -> Delay9/1, pilotIdx/1
  RRC Receive Matched Filter/1 -> Symbol Synchronizer/1(dataIn)
  Delay8/1 -> Coarse Frequency Estimator/3(pilotValid)
  Delay3/1 -> Product/1
  Delay6/1 -> Math Function/1
  Delay11/1 -> Delay34/1
  Delay14/1 -> RRC Receive Matched Filter/1
  Delay5/1 -> Delay2/1
  Product/1 -> Delay14/1
  Delay2/1 -> Product/2
  validIn/1 -> Delay1/1
  Delay29/1 -> Delay8/1, pilotValid/1
  RRC Receive Matched Filter/2 -> Symbol Synchronizer/2(validIn)
  PL Data Descrambler and Pilot Valid Indicator/4(validOut) -> Delay31/1
  Delay10/1 -> Delay11/1
  PL Data Descrambler and Pilot Valid Indicator/2(pilotValid) -> Delay29/1
  Delay9/1 -> Coarse Frequency Estimator/4(pilotIdx)
  Symbol Synchronizer/2(validOut) -> symbSyncValidOut/1, Frame Synchronizer/2(validIn)
  dataIn/1 -> Delay3/1
  Frame Synchronizer/4(hasPilots) -> PL Data Descrambler and Pilot Valid Indicator/4(hasPilots), Delay10/1
  Delay1/1 -> Delay4/1
  Frame Synchronizer/1(dataOut) -> PL Data Descrambler and Pilot Valid Indicator/1(dataIn)
  Frame Synchronizer/5(VisualizeCorrelationSignals) -> VisualizeCorrelationSignals/1
  rstCCFO/1 -> Coarse Frequency Estimator/1(rst)

== system soc_dvbs2_fpga/DVBS2/DVBS2 TxRx/DVB-S2 HDL Receiver/Synchronizer and PL Header Decoder/Time Frequency and Coarse Phase Synchronizer/Variance Estimator ==
  pilotValid : Inport
  dataIn : Inport  Port=2
  validIn : Inport  Port=3
  endOfSOFIn : Inport  Port=4
  Add : Sum  Inputs=+-  OutDataTypeStr=Inherit: Same as first input
  Complex to Real-Imag : ComplexToRealImag  Output=Real
  Constant : Constant  Value=fi(config.Pilot,1,18,13)  SampleTime=-1
  Constant1 : Constant  Value=complex(0)  OutDataTypeStr=Inherit: Inherit via back propagation  SampleTime=-1
  Data Type Conversion : DataTypeConversion  OutDataTypeStr=fixdt(1,30,18)  SaturateOnIntegerOverflow=off  RndMeth=Floor
  Delay{1,5..6,9..16} (11 alike) : Delay
  Delay{2..4,7..8,17..26} (15 alike) : Delay  DelayLength=1
  Delay27 : Delay  DelayLength=4
  Delay28 : Delay  DelayLength=4
  Delay29 : Delay  DelayLength=4
  Math Function : Math  Operator=conj
  "Moving Average " : Subsystem
  Product : Product
  Switch : Switch  Criteria=u2 > Threshold  SaturateOnIntegerOverflow=off  InputSameDT=off
  dataOut : Outport
  validOut : Outport  Port=2
  endOfSOF : Outport  Port=3
  varOut : Outport  Port=4
  wires:
  Delay8/1 -> Switch/1
  Constant1/1 -> Switch/3
  Switch/1 -> Add/2
  Constant/1 -> Delay8/1
  Data Type Conversion/1 -> Complex to Real-Imag/1
  Delay17/1 -> Math Function/1, Delay1/1
  Product/1 -> Delay5/1
  Add/1 -> Delay17/1
  Delay29/1 -> endOfSOF/1
  Delay28/1 -> validOut/1
  Delay27/1 -> dataOut/1
  Delay26/1 -> Delay29/1
  Delay25/1 -> Delay28/1
  Delay24/1 -> Delay27/1
  Delay23/1 -> "Moving Average "/1(enable)
  Delay22/1 -> "Moving Average "/2(dataIn)
  Delay21/1 -> Delay9/1
  Delay20/1 -> Delay15/1
  Delay19/1 -> Delay14/1
  Delay18/1 -> Delay11/1
  Delay16/1 -> Delay26/1
  Delay15/1 -> Delay16/1
  Delay14/1 -> Delay13/1
  Delay13/1 -> Delay25/1
  Delay12/1 -> Delay24/1
  Delay11/1 -> Delay12/1
  Delay10/1 -> Delay23/1
  Delay9/1 -> Delay10/1
  Delay6/1 -> Product/2
  Delay5/1 -> Data Type Conversion/1
  Delay1/1 -> Product/1
  "Moving Average "/1(avgOut) -> varOut/1
  Delay7/1 -> Delay21/1, Switch/2
  Complex to Real-Imag/1 -> Delay22/1
  Math Function/1 -> Delay6/1
  endOfSOFIn/1 -> Delay2/1
  dataIn/1 -> Delay4/1
  validIn/1 -> Delay3/1
  pilotValid/1 -> Delay7/1
  Delay3/1 -> Delay19/1
  Delay2/1 -> Delay20/1
  Delay4/1 -> Delay18/1, Add/1

== system soc_dvbs2_fpga/DVBS2/DVBS2 TxRx/LUT Based Tx/Subsystem1/Subsystem/txLUT1 ==
  rst : Inport
  enb : Inport  Port=2
  1-D Lookup Table : Lookup_n-D  NumberOfTableDimensions=1  BreakpointsSpecification=Even spacing  BreakpointsForDimension1=0:length(txDataOut)-1  BreakpointsForDimension1FirstPoint=0  Table=fi(DataLUT,1,18,16)  TableDataTypeStr=Inherit: Inherit from 'Table data'  InterpMethod=Flat  InternalRulePriority=Speed  OutDataTypeStr=Inherit: Inherit from 'Table data'  RndMeth=Simplest
  Compare To Constant : simulink/Logic and Bit Operations/Compare To Constant  relop===  const=length(DataLUT) - 2  OutDataTypeStr=boolean
  HDL Counter : hdlsllib/Sources/HDL Counter  CountType=Count limited  CountInit=0  CountStep=1  CountMax=length(DataLUT)-1  CountFromType=Initial value  CountFrom=0  CountResetPort=on  CountLoadPort=off  CountEnbPort=on  CountDirPort=off  CountHitOutputPort=off  CountDataType=Unsigned  CountWordLen=nextpow2(length(DataLUT)-1)  CountFracLen=0  CountSampTime=1
  Out1 : Outport
  endOfLUT : Outport  Port=2
  wires:
  1-D Lookup Table/1 -> Out1/1
  HDL Counter/1 -> Compare To Constant/1, 1-D Lookup Table/1
  enb/1 -> HDL Counter/2
  Compare To Constant/1 -> endOfLUT/1
  rst/1 -> HDL Counter/1

== system soc_dvbs2_fpga/DVBS2/DVBS2 TxRx/LUT Based Tx/Subsystem1/Subsystem/txLUT2 ==
  rst : Inport
  enb : Inport  Port=2
  1-D Lookup Table : Lookup_n-D  NumberOfTableDimensions=1  BreakpointsSpecification=Even spacing  BreakpointsForDimension1=0:length(txDataOut)-1  BreakpointsForDimension1FirstPoint=0  Table=fi(DataLUT,1,18,16)  TableDataTypeStr=Inherit: Inherit from 'Table data'  InterpMethod=Flat  InternalRulePriority=Speed  OutDataTypeStr=Inherit: Inherit from 'Table data'  RndMeth=Simplest
  Compare To Constant : simulink/Logic and Bit Operations/Compare To Constant  relop===  const=length(DataLUT) - 2  OutDataTypeStr=boolean
  HDL Counter : hdlsllib/Sources/HDL Counter  CountType=Count limited  CountInit=0  CountStep=1  CountMax=length(DataLUT)-1  CountFromType=Initial value  CountFrom=0  CountResetPort=on  CountLoadPort=off  CountEnbPort=on  CountDirPort=off  CountHitOutputPort=off  CountDataType=Unsigned  CountWordLen=nextpow2(length(DataLUT)-1)  CountFracLen=0  CountSampTime=1
  Out1 : Outport
  endOfLUT : Outport  Port=2
  wires:
  rst/1 -> HDL Counter/1
  Compare To Constant/1 -> endOfLUT/1
  enb/1 -> HDL Counter/2
  HDL Counter/1 -> 1-D Lookup Table/1, Compare To Constant/1
  1-D Lookup Table/1 -> Out1/1

== system soc_dvbs2_fpga/DVBS2/DVBS2 TxRx/LUT Based Tx/Subsystem1/Subsystem/txLUT3 ==
  rst : Inport
  enb : Inport  Port=2
  1-D Lookup Table : Lookup_n-D  NumberOfTableDimensions=1  BreakpointsSpecification=Even spacing  BreakpointsForDimension1=0:length(txDataOut)-1  BreakpointsForDimension1FirstPoint=0  Table=fi(DataLUT,1,18,16)  TableDataTypeStr=Inherit: Inherit from 'Table data'  InterpMethod=Flat  InternalRulePriority=Speed  OutDataTypeStr=Inherit: Inherit from 'Table data'  RndMeth=Simplest
  Compare To Constant : simulink/Logic and Bit Operations/Compare To Constant  relop===  const=length(DataLUT) - 2  OutDataTypeStr=boolean
  HDL Counter : hdlsllib/Sources/HDL Counter  CountType=Count limited  CountInit=0  CountStep=1  CountMax=length(DataLUT)-1  CountFromType=Initial value  CountFrom=0  CountResetPort=on  CountLoadPort=off  CountEnbPort=on  CountDirPort=off  CountHitOutputPort=off  CountDataType=Unsigned  CountWordLen=nextpow2(length(DataLUT)-1)  CountFracLen=0  CountSampTime=1
  Out1 : Outport
  endOfLUT : Outport  Port=2
  wires:
  rst/1 -> HDL Counter/1
  Compare To Constant/1 -> endOfLUT/1
  enb/1 -> HDL Counter/2
  HDL Counter/1 -> 1-D Lookup Table/1, Compare To Constant/1
  1-D Lookup Table/1 -> Out1/1

== system soc_dvbs2_fpga/DVBS2/DVBS2 TxRx/LUT Based Tx/Subsystem1/Subsystem/txLUT4 ==
  rst : Inport
  enb : Inport  Port=2
  1-D Lookup Table : Lookup_n-D  NumberOfTableDimensions=1  BreakpointsSpecification=Even spacing  BreakpointsForDimension1=0:length(txDataOut)-1  BreakpointsForDimension1FirstPoint=0  Table=fi(DataLUT,1,18,16)  TableDataTypeStr=Inherit: Inherit from 'Table data'  InterpMethod=Flat  InternalRulePriority=Speed  OutDataTypeStr=Inherit: Inherit from 'Table data'  RndMeth=Simplest
  Compare To Constant : simulink/Logic and Bit Operations/Compare To Constant  relop===  const=length(DataLUT) - 2  OutDataTypeStr=boolean
  HDL Counter : hdlsllib/Sources/HDL Counter  CountType=Count limited  CountInit=0  CountStep=1  CountMax=length(DataLUT)-1  CountFromType=Initial value  CountFrom=0  CountResetPort=on  CountLoadPort=off  CountEnbPort=on  CountDirPort=off  CountHitOutputPort=off  CountDataType=Unsigned  CountWordLen=nextpow2(length(DataLUT)-1)  CountFracLen=0  CountSampTime=1
  Out1 : Outport
  endOfLUT : Outport  Port=2
  wires:
  1-D Lookup Table/1 -> Out1/1
  HDL Counter/1 -> Compare To Constant/1, 1-D Lookup Table/1
  enb/1 -> HDL Counter/2
  Compare To Constant/1 -> endOfLUT/1
  rst/1 -> HDL Counter/1

== system soc_dvbs2_fpga/DVBS2/DVBS2 TxRx/LUT Based Tx/Subsystem1/Subsystem/txLUT5 ==
  rst : Inport
  enb : Inport  Port=2
  1-D Lookup Table : Lookup_n-D  NumberOfTableDimensions=1  BreakpointsSpecification=Even spacing  BreakpointsForDimension1=0:length(txDataOut)-1  BreakpointsForDimension1FirstPoint=0  Table=fi(DataLUT,1,18,16)  TableDataTypeStr=Inherit: Inherit from 'Table data'  InterpMethod=Flat  InternalRulePriority=Speed  OutDataTypeStr=Inherit: Inherit from 'Table data'  RndMeth=Simplest
  Compare To Constant : simulink/Logic and Bit Operations/Compare To Constant  relop===  const=length(DataLUT) - 2  OutDataTypeStr=boolean
  HDL Counter : hdlsllib/Sources/HDL Counter  CountType=Count limited  CountInit=0  CountStep=1  CountMax=length(DataLUT)-1  CountFromType=Initial value  CountFrom=0  CountResetPort=on  CountLoadPort=off  CountEnbPort=on  CountDirPort=off  CountHitOutputPort=off  CountDataType=Unsigned  CountWordLen=nextpow2(length(DataLUT)-1)  CountFracLen=0  CountSampTime=1
  Out1 : Outport
  endOfLUT : Outport  Port=2
  wires:
  rst/1 -> HDL Counter/1
  Compare To Constant/1 -> endOfLUT/1
  enb/1 -> HDL Counter/2
  HDL Counter/1 -> 1-D Lookup Table/1, Compare To Constant/1
  1-D Lookup Table/1 -> Out1/1

== system soc_dvbs2_fpga/DVBS2/DVBS2 TxRx/LUT Based Tx/Subsystem1/Subsystem/txLUT6 ==
  rst : Inport
  enb : Inport  Port=2
  1-D Lookup Table : Lookup_n-D  NumberOfTableDimensions=1  BreakpointsSpecification=Even spacing  BreakpointsForDimension1=0:length(txDataOut)-1  BreakpointsForDimension1FirstPoint=0  Table=fi(DataLUT,1,18,16)  TableDataTypeStr=Inherit: Inherit from 'Table data'  InterpMethod=Flat  InternalRulePriority=Speed  OutDataTypeStr=Inherit: Inherit from 'Table data'  RndMeth=Simplest
  Compare To Constant : simulink/Logic and Bit Operations/Compare To Constant  relop===  const=length(DataLUT) - 2  OutDataTypeStr=boolean
  HDL Counter : hdlsllib/Sources/HDL Counter  CountType=Count limited  CountInit=0  CountStep=1  CountMax=length(DataLUT)-1  CountFromType=Initial value  CountFrom=0  CountResetPort=on  CountLoadPort=off  CountEnbPort=on  CountDirPort=off  CountHitOutputPort=off  CountDataType=Unsigned  CountWordLen=nextpow2(length(DataLUT)-1)  CountFracLen=0  CountSampTime=1
  Out1 : Outport
  endOfLUT : Outport  Port=2
  wires:
  1-D Lookup Table/1 -> Out1/1
  HDL Counter/1 -> Compare To Constant/1, 1-D Lookup Table/1
  enb/1 -> HDL Counter/2
  Compare To Constant/1 -> endOfLUT/1
  rst/1 -> HDL Counter/1

== system soc_dvbs2_fpga/DVBS2/DVBS2 TxRx/LUT Based Tx/Subsystem1/Subsystem1/txLUT1 ==
  rst : Inport
  enb : Inport  Port=2
  1-D Lookup Table : Lookup_n-D  NumberOfTableDimensions=1  BreakpointsSpecification=Even spacing  BreakpointsForDimension1=0:length(txDataOut)-1  BreakpointsForDimension1FirstPoint=0  Table=fi(DataLUT,1,18,16)  TableDataTypeStr=Inherit: Inherit from 'Table data'  InterpMethod=Flat  InternalRulePriority=Speed  OutDataTypeStr=Inherit: Inherit from 'Table data'  RndMeth=Simplest
  Compare To Constant : simulink/Logic and Bit Operations/Compare To Constant  relop===  const=length(DataLUT) - 2  OutDataTypeStr=boolean
  HDL Counter : hdlsllib/Sources/HDL Counter  CountType=Count limited  CountInit=0  CountStep=1  CountMax=length(DataLUT)-1  CountFromType=Initial value  CountFrom=0  CountResetPort=on  CountLoadPort=off  CountEnbPort=on  CountDirPort=off  CountHitOutputPort=off  CountDataType=Unsigned  CountWordLen=nextpow2(length(DataLUT)-1)  CountFracLen=0  CountSampTime=1
  Out1 : Outport
  endOfLUT : Outport  Port=2
  wires:
  rst/1 -> HDL Counter/1
  Compare To Constant/1 -> endOfLUT/1
  enb/1 -> HDL Counter/2
  HDL Counter/1 -> 1-D Lookup Table/1, Compare To Constant/1
  1-D Lookup Table/1 -> Out1/1

== system soc_dvbs2_fpga/DVBS2/DVBS2 TxRx/LUT Based Tx/Subsystem1/Subsystem1/txLUT2 ==
  rst : Inport
  enb : Inport  Port=2
  1-D Lookup Table : Lookup_n-D  NumberOfTableDimensions=1  BreakpointsSpecification=Even spacing  BreakpointsForDimension1=0:length(txDataOut)-1  BreakpointsForDimension1FirstPoint=0  Table=fi(DataLUT,1,18,16)  TableDataTypeStr=Inherit: Inherit from 'Table data'  InterpMethod=Flat  InternalRulePriority=Speed  OutDataTypeStr=Inherit: Inherit from 'Table data'  RndMeth=Simplest
  Compare To Constant : simulink/Logic and Bit Operations/Compare To Constant  relop===  const=length(DataLUT) - 2  OutDataTypeStr=boolean
  HDL Counter : hdlsllib/Sources/HDL Counter  CountType=Count limited  CountInit=0  CountStep=1  CountMax=length(DataLUT)-1  CountFromType=Initial value  CountFrom=0  CountResetPort=on  CountLoadPort=off  CountEnbPort=on  CountDirPort=off  CountHitOutputPort=off  CountDataType=Unsigned  CountWordLen=nextpow2(length(DataLUT)-1)  CountFracLen=0  CountSampTime=1
  Out1 : Outport
  endOfLUT : Outport  Port=2
  wires:
  1-D Lookup Table/1 -> Out1/1
  HDL Counter/1 -> Compare To Constant/1, 1-D Lookup Table/1
  enb/1 -> HDL Counter/2
  Compare To Constant/1 -> endOfLUT/1
  rst/1 -> HDL Counter/1

== system soc_dvbs2_fpga/DVBS2/DVBS2 TxRx/LUT Based Tx/Subsystem1/Subsystem1/txLUT3 ==
  rst : Inport
  enb : Inport  Port=2
  1-D Lookup Table : Lookup_n-D  NumberOfTableDimensions=1  BreakpointsSpecification=Even spacing  BreakpointsForDimension1=0:length(txDataOut)-1  BreakpointsForDimension1FirstPoint=0  Table=fi(DataLUT,1,18,16)  TableDataTypeStr=Inherit: Inherit from 'Table data'  InterpMethod=Flat  InternalRulePriority=Speed  OutDataTypeStr=Inherit: Inherit from 'Table data'  RndMeth=Simplest
  Compare To Constant : simulink/Logic and Bit Operations/Compare To Constant  relop===  const=length(DataLUT) - 2  OutDataTypeStr=boolean
  HDL Counter : hdlsllib/Sources/HDL Counter  CountType=Count limited  CountInit=0  CountStep=1  CountMax=length(DataLUT)-1  CountFromType=Initial value  CountFrom=0  CountResetPort=on  CountLoadPort=off  CountEnbPort=on  CountDirPort=off  CountHitOutputPort=off  CountDataType=Unsigned  CountWordLen=nextpow2(length(DataLUT)-1)  CountFracLen=0  CountSampTime=1
  Out1 : Outport
  endOfLUT : Outport  Port=2
  wires:
  1-D Lookup Table/1 -> Out1/1
  HDL Counter/1 -> Compare To Constant/1, 1-D Lookup Table/1
  enb/1 -> HDL Counter/2
  Compare To Constant/1 -> endOfLUT/1
  rst/1 -> HDL Counter/1

== system soc_dvbs2_fpga/DVBS2/DVBS2 TxRx/LUT Based Tx/Subsystem1/Subsystem1/txLUT4 ==
  rst : Inport
  enb : Inport  Port=2
  1-D Lookup Table : Lookup_n-D  NumberOfTableDimensions=1  BreakpointsSpecification=Even spacing  BreakpointsForDimension1=0:length(txDataOut)-1  BreakpointsForDimension1FirstPoint=0  Table=fi(DataLUT,1,18,16)  TableDataTypeStr=Inherit: Inherit from 'Table data'  InterpMethod=Flat  InternalRulePriority=Speed  OutDataTypeStr=Inherit: Inherit from 'Table data'  RndMeth=Simplest
  Compare To Constant : simulink/Logic and Bit Operations/Compare To Constant  relop===  const=length(DataLUT) - 1  OutDataTypeStr=boolean
  HDL Counter : hdlsllib/Sources/HDL Counter  CountType=Count limited  CountInit=0  CountStep=1  CountMax=length(DataLUT)-1  CountFromType=Initial value  CountFrom=0  CountResetPort=on  CountLoadPort=off  CountEnbPort=on  CountDirPort=off  CountHitOutputPort=off  CountDataType=Unsigned  CountWordLen=nextpow2(length(DataLUT)-1)  CountFracLen=0  CountSampTime=1
  Out1 : Outport
  endOfLUT : Outport  Port=2
  wires:
  rst/1 -> HDL Counter/1
  Compare To Constant/1 -> endOfLUT/1
  enb/1 -> HDL Counter/2
  HDL Counter/1 -> 1-D Lookup Table/1, Compare To Constant/1
  1-D Lookup Table/1 -> Out1/1
